simulink model "GuidanSim"  (R2024b)
settings: Solver=FixedStepAuto  StartTime=0.0  StopTime=inf  RelTol=1e-3
values from neighbouring files (symbols this model uses):
  gM = deg2rad(30)    [GuidanceSimParams.m]
  N = 2    [GuidanceSimParams.m]
  Rlethal = 1    [GuidanceSimParams.m]
  RM = [xM;zM]    [GuidanceSimParams.m]
  RT = [xT;zT]    [GuidanceSimParams.m]
  VM = [600*cos(gM),-600*sin(gM)]    [GuidanceSimParams.m]
  VT = [400*cos(gT),-400*sin(gT)]    [GuidanceSimParams.m]
libraries: simulink_extras x3, simulink x2, aerolibanim x1
settings Model: Creator=Ameya  LastModifiedBy=Ameya

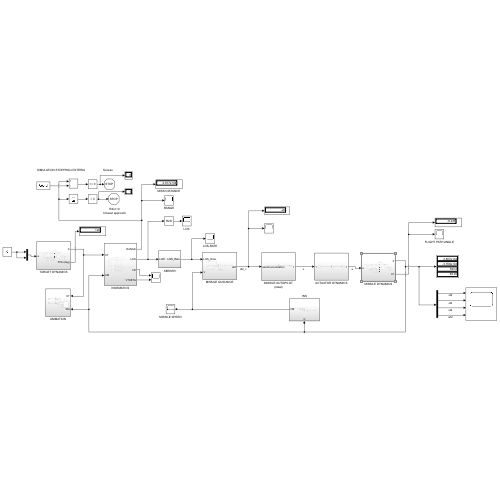
[thumbnail: Simulink's stored preview of the top-level diagram]
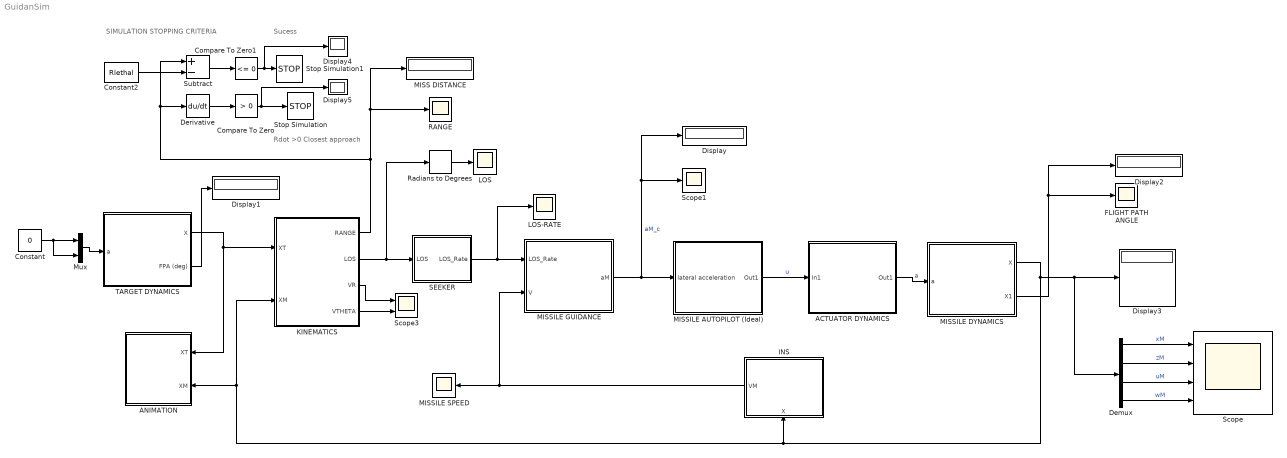
== system GuidanSim ==
  note: Rdot >0
      | Closest approach
  note: SIMULATION STOPPING CRITERIA
  note: Sucess
  ACTUATOR DYNAMICS : Subsystem
  ANIMATION : Subsystem
  Compare To Zero : simulink/Logic and Bit Operations/Compare To Zero  relop=>  OutDataTypeStr=boolean
  Compare To Zero1 : simulink/Logic and Bit Operations/Compare To Zero  relop=<=  OutDataTypeStr=boolean
  Constant : Constant  Value=0
  Constant2 : Constant  Value=Rlethal
  Demux : Demux
  Derivative : Derivative
  Display{,1..5} (6 alike) : Display
  FLIGHT PATH ANGLE : Scope
  INS : Subsystem
      settings: PortSchema="{\"entries\":[{\"content\":{\"sides\":[{\"content\":{},\"type\":\"ConnectorPlacement.EquallySpacedRectSide\",\"uuid\":\"3a75d8bd-203c-4ca4-9f28-a00dd574f861\"},{\"content\":{\"connectorIds\":[\"Out1\"],\"side\":\"RIGHT\"},\"type\":\"ConnectorPlacement.EquallySpacedRectSide\",\"uuid\":\"f6d8c757-0e96-437e-9198-94cbd887d432\"},{\"content\":{\"side\":\"TOP\"},\"type\":\"ConnectorPlacement.EquallySpacedRectSide\",\"uuid\":\"41075b2e-5d18-45ea-a6fc-7f66ef6598ab\"},{\"content\":{\"connectorIds\":[\"In1\"],\"side\":\"BOTTOM\"},\"type\":\"ConnectorPlacement.EquallySpacedRectSide\",\"uuid\":\"891ca2b5-b4ab-4086-9ff4-c4d2df822072\"}]},\"type\":\"ConnectorPlacement.EquallySpacedConnector\",\"uuid\":\"9a7247ef-0899-430c-baeb-b82ca1b0d294\"}],\"packageUris\":[\"http://schema.mathworks.com/mf0/Connector/R2020b\"],\"version\":\"1.0\"}"
  KINEMATICS : Subsystem
  LOS : Scope
  LOS-RATE : Scope
  MISS DISTANCE : Display
  MISSILE AUTOPILOT (Ideal) : Subsystem
  MISSILE DYNAMICS : Subsystem
  MISSILE GUIDANCE : Subsystem
  MISSILE SPEED : Scope
  Mux : Mux  Inputs=2
  RANGE : Scope
  Radians to Degrees : simulink_extras/Transformations/Radians to Degrees
  SEEKER : Subsystem
  Scope : Scope  NumInputPorts=4
  Scope1 : Scope
  Scope3 : Scope  NumInputPorts=2
  Stop Simulation : Stop
  Stop Simulation1 : Stop
  Subtract : Sum  Inputs=+-
  TARGET DYNAMICS : Subsystem
  wires:
  MISSILE AUTOPILOT (Ideal)/1(Out1) -> ACTUATOR DYNAMICS/1(In1)  "u"
  MISSILE GUIDANCE/1(aM) -> Scope1/1, Display/1, MISSILE AUTOPILOT (Ideal)/1(lateral acceleration)  "aM_c"
  ACTUATOR DYNAMICS/1(Out1) -> MISSILE DYNAMICS/1(a)  "a"
  MISSILE DYNAMICS/1(X) -> Demux/1, Display3/1, KINEMATICS/2(XM), ANIMATION/2(XM), INS/1(X)
  TARGET DYNAMICS/1(X) -> KINEMATICS/1(XT), ANIMATION/1(XT)
  SEEKER/1(LOS_Rate) -> LOS-RATE/1, MISSILE GUIDANCE/1(LOS_Rate)
  Constant/1 -> Mux/2, Mux/1
  Mux/1 -> TARGET DYNAMICS/1(a)
  KINEMATICS/2(LOS) -> Radians to Degrees/1, SEEKER/1(LOS)
  Radians to Degrees/1 -> LOS/1
  Compare To Zero/1 -> Display5/1, Stop Simulation/1
  Derivative/1 -> Compare To Zero/1
  KINEMATICS/1(RANGE) -> MISS DISTANCE/1, RANGE/1, Subtract/1, Derivative/1
  Constant2/1 -> Subtract/2
  Subtract/1 -> Compare To Zero1/1
  Compare To Zero1/1 -> Display4/1, Stop Simulation1/1
  INS/1(VM) -> MISSILE GUIDANCE/2(V), MISSILE SPEED/1
  Demux/1 -> Scope/1  "xM"
  Demux/2 -> Scope/2  "zM"
  Demux/3 -> Scope/3  "uM"
  Demux/4 -> Scope/4  "wM"
  KINEMATICS/3(VR) -> Scope3/1
  KINEMATICS/4(VTHETA) -> Scope3/2
  TARGET DYNAMICS/2(FPA (deg)) -> Display1/1
  MISSILE DYNAMICS/2(X1) -> Display2/1, FLIGHT PATH ANGLE/1

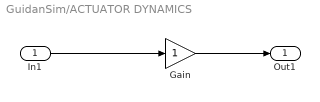
== system GuidanSim/ACTUATOR DYNAMICS ==
  In1 : Inport
  Gain : Gain
  Out1 : Outport
  wires:
  In1/1 -> Gain/1
  Gain/1 -> Out1/1

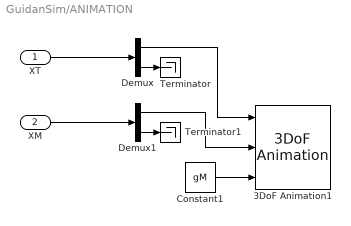
== system GuidanSim/ANIMATION ==
  XT : Inport
  XM : Inport  Port=2
  3DoF Animation1 : aerolibanim/3DoF Animation  u1=[0 5000 -2000 2000 -5050 -3]  u2=0.05  u3=5  u5=Fixed position  u6=[2000 500 -3150]  u7=10  u8=on
  Constant1 : Constant  Value=gM
  Demux : Demux  Outputs=2
  Demux1 : Demux  Outputs=2
  Terminator : Terminator
  Terminator1 : Terminator
  wires:
  Demux1/1 -> 3DoF Animation1/2
  XT/1 -> Demux/1
  Constant1/1 -> 3DoF Animation1/3
  Demux1/2 -> Terminator1/1
  Demux/1 -> 3DoF Animation1/1
  Demux/2 -> Terminator/1
  XM/1 -> Demux1/1

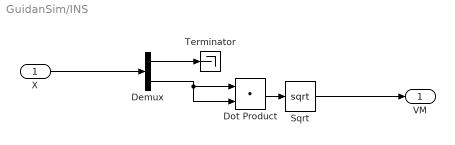
== system GuidanSim/INS ==
  X : Inport
  Demux : Demux  Outputs=2
  Dot Product : DotProduct  OutDataTypeStr=Inherit: Inherit via internal rule
  Sqrt : Sqrt
  Terminator : Terminator
  VM : Outport
  wires:
  X/1 -> Demux/1
  Demux/1 -> Terminator/1
  Dot Product/1 -> Sqrt/1
  Demux/2 -> Dot Product/1, Dot Product/2
  Sqrt/1 -> VM/1

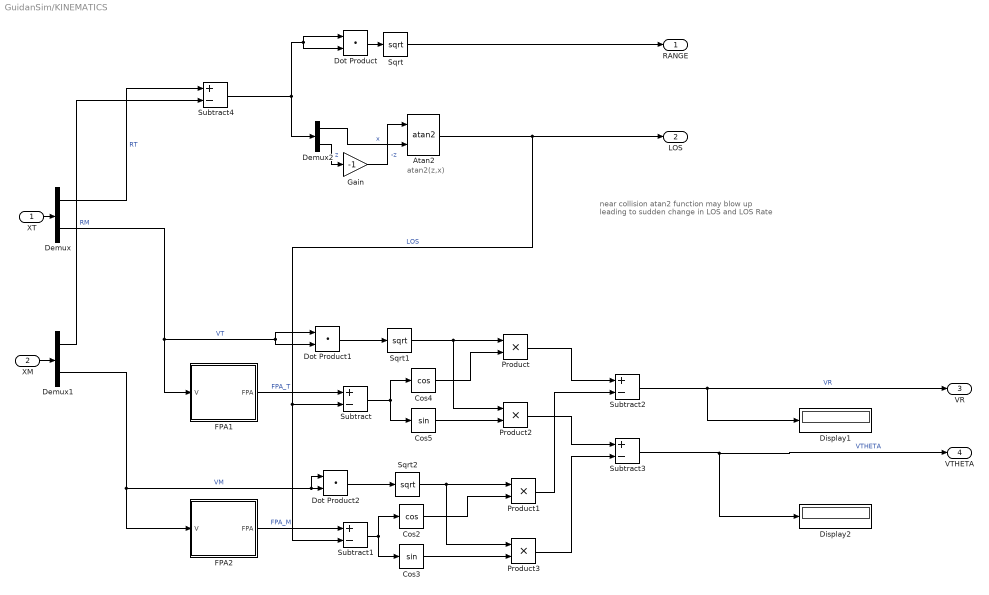
== system GuidanSim/KINEMATICS ==
  note: near collision atan2 function may blow up
      | leading to sudden change in LOS and LOS Rate
  note: atan2(z,x)
  XT : Inport
  XM : Inport  Port=2
  Atan2 : Trigonometry  Operator=atan2
  Cos2 : Trigonometry  Operator=cos
  Cos3 : Trigonometry
  Cos4 : Trigonometry  Operator=cos
  Cos5 : Trigonometry
  Demux : Demux  Outputs=2
  Demux1 : Demux  Outputs=2
  Demux2 : Demux  Outputs=2
  Display1 : Display
  Display2 : Display
  Dot Product : DotProduct  OutDataTypeStr=Inherit: Inherit via internal rule
  Dot Product1 : DotProduct  OutDataTypeStr=Inherit: Inherit via internal rule
  Dot Product2 : DotProduct  OutDataTypeStr=Inherit: Inherit via internal rule
  FPA1 : Subsystem
  FPA2 : Subsystem
  Gain : Gain  Gain=-1
  Product{,1..3} (4 alike) : Product
  Sqrt : Sqrt
  Sqrt1 : Sqrt
  Sqrt2 : Sqrt
  Subtract{,1..4} (5 alike) : Sum  Inputs=+-
  RANGE : Outport
  LOS : Outport  Port=2
  VR : Outport  Port=3
  VTHETA : Outport  Port=4
  wires:
  XT/1 -> Demux/1
  XM/1 -> Demux1/1
  Atan2/1 -> LOS/1, Subtract/2, Subtract1/2  "LOS"
  Demux/1 -> Subtract4/1  "RT"
  Demux1/1 -> Subtract4/2  "RM"
  Demux/2 -> Dot Product1/1, Dot Product1/2, FPA1/1(V)  "VT"
  FPA1/1(FPA) -> Subtract/1  "FPA_T"
  FPA2/1(FPA) -> Subtract1/1  "FPA_M"
  Subtract1/1 -> Cos3/1, Cos2/1
  Subtract/1 -> Cos5/1, Cos4/1
  Dot Product1/1 -> Sqrt1/1
  Sqrt1/1 -> Product2/1, Product/1
  Cos4/1 -> Product/2
  Sqrt2/1 -> Product3/1, Product1/1
  Demux1/2 -> Dot Product2/1, Dot Product2/2, FPA2/1(V)  "VM"
  Dot Product2/1 -> Sqrt2/1
  Cos2/1 -> Product1/2
  Product/1 -> Subtract2/1
  Product1/1 -> Subtract2/2
  Subtract2/1 -> VR/1, Display1/1  "VR"
  Subtract3/1 -> VTHETA/1, Display2/1  "VTHETA"
  Cos5/1 -> Product2/2
  Cos3/1 -> Product3/2
  Product3/1 -> Subtract3/2
  Product2/1 -> Subtract3/1
  Sqrt/1 -> RANGE/1
  Dot Product/1 -> Sqrt/1
  Gain/1 -> Atan2/1  "-z"
  Demux2/2 -> Gain/1  "z"
  Demux2/1 -> Atan2/2  "x"
  Subtract4/1 -> Dot Product/1, Dot Product/2, Demux2/1

== system GuidanSim/MISSILE AUTOPILOT (Ideal) ==
  lateral acceleration : Inport
  Gain : Gain
  Out1 : Outport
  wires:
  lateral acceleration/1 -> Gain/1
  Gain/1 -> Out1/1

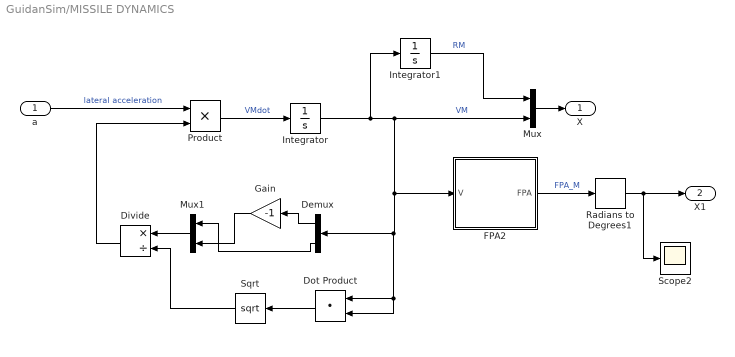
== system GuidanSim/MISSILE DYNAMICS ==
  a : Inport
  Demux : Demux  Outputs=2
  Divide : Product  Inputs=*/
  Dot Product : DotProduct  OutDataTypeStr=Inherit: Inherit via internal rule
  FPA2 : Subsystem
  Gain : Gain  Gain=-1
  Integrator : Integrator  InitialCondition=VM  UpperSaturationLimit=VM  LowerSaturationLimit=VM-0.000001
  Integrator1 : Integrator  InitialCondition=RM
  Mux : Mux  Inputs=2
  Mux1 : Mux  Inputs=2
  Product : Product
  Radians to Degrees1 : simulink_extras/Transformations/Radians to Degrees
  Scope2 : Scope
  Sqrt : Sqrt
  X : Outport
  X1 : Outport  Port=2
  wires:
  Integrator/1 -> Integrator1/1, FPA2/1(V), Dot Product/2, Dot Product/1, Demux/1, Mux/2  "VM"
  Integrator1/1 -> Mux/1  "RM"
  Mux/1 -> X/1
  Demux/1 -> Gain/1
  Gain/1 -> Mux1/2
  Demux/2 -> Mux1/1
  Dot Product/1 -> Sqrt/1
  a/1 -> Product/1  "lateral acceleration"
  Product/1 -> Integrator/1  "VMdot"
  Mux1/1 -> Divide/1
  Sqrt/1 -> Divide/2
  Divide/1 -> Product/2
  Radians to Degrees1/1 -> X1/1, Scope2/1
  FPA2/1(FPA) -> Radians to Degrees1/1  "FPA_M"

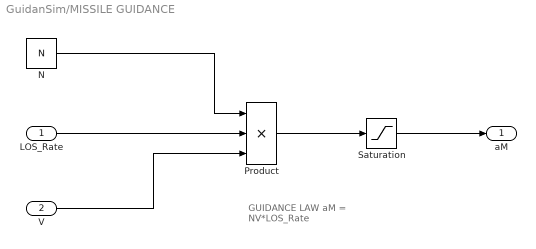
== system GuidanSim/MISSILE GUIDANCE ==
  note: GUIDANCE LAW
      | aM = NV*LOS_Rate
  LOS_Rate : Inport
  V : Inport  Port=2
  N : Constant  Value=N
  Product : Product  Inputs=3
  Saturation : Saturate  UpperLimit=+20  LowerLimit=-20
  aM : Outport
  wires:
  N/1 -> Product/1
  Product/1 -> Saturation/1
  LOS_Rate/1 -> Product/2
  V/1 -> Product/3
  Saturation/1 -> aM/1

== system GuidanSim/SEEKER ==
  LOS : Inport
  Derivative : Derivative
  LOS_Rate : Outport
  wires:
  LOS/1 -> Derivative/1
  Derivative/1 -> LOS_Rate/1

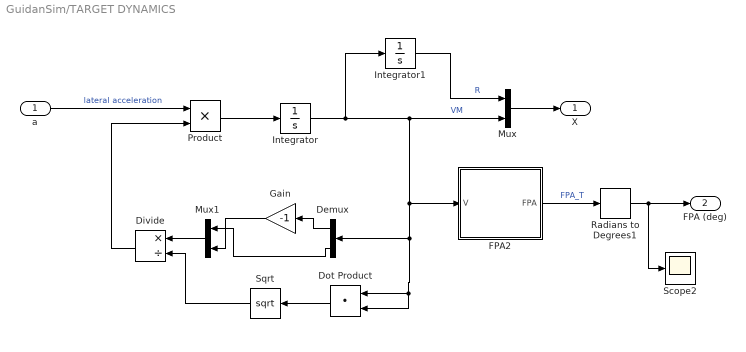
== system GuidanSim/TARGET DYNAMICS ==
  a : Inport
  Demux : Demux  Outputs=2
  Divide : Product  Inputs=*/
  Dot Product : DotProduct  OutDataTypeStr=Inherit: Inherit via internal rule
  FPA2 : Subsystem
  Gain : Gain  Gain=-1
  Integrator : Integrator  InitialCondition=VT
  Integrator1 : Integrator  InitialCondition=RT
  Mux : Mux  Inputs=2
  Mux1 : Mux  Inputs=2
  Product : Product
  Radians to Degrees1 : simulink_extras/Transformations/Radians to Degrees
  Scope2 : Scope
  Sqrt : Sqrt
  X : Outport
  FPA (deg) : Outport  Port=2
  wires:
  a/1 -> Product/1  "lateral acceleration"
  Integrator1/1 -> Mux/1  "R"
  Mux/1 -> X/1
  Demux/2 -> Mux1/1
  Dot Product/1 -> Sqrt/1
  Demux/1 -> Gain/1
  Sqrt/1 -> Divide/2
  Divide/1 -> Product/2
  Mux1/1 -> Divide/1
  Gain/1 -> Mux1/2
  Product/1 -> Integrator/1
  Integrator/1 -> Integrator1/1, FPA2/1(V), Dot Product/2, Dot Product/1, Demux/1, Mux/2  "VM"
  Radians to Degrees1/1 -> FPA (deg)/1, Scope2/1
  FPA2/1(FPA) -> Radians to Degrees1/1  "FPA_T"

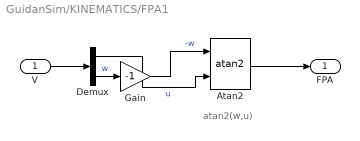
== system GuidanSim/KINEMATICS/FPA1 ==
  note: atan2(w,u)
  V : Inport
  Atan2 : Trigonometry  Operator=atan2
  Demux : Demux  Outputs=2
  Gain : Gain  Gain=-1
  FPA : Outport
  wires:
  V/1 -> Demux/1
  Demux/2 -> Gain/1  "w"
  Demux/1 -> Atan2/2  "u"
  Atan2/1 -> FPA/1
  Gain/1 -> Atan2/1  "-w"

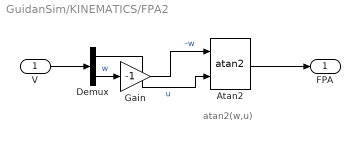
== system GuidanSim/KINEMATICS/FPA2 ==
  note: atan2(w,u)
  V : Inport
  Atan2 : Trigonometry  Operator=atan2
  Demux : Demux  Outputs=2
  Gain : Gain  Gain=-1
  FPA : Outport
  wires:
  V/1 -> Demux/1
  Demux/2 -> Gain/1  "w"
  Demux/1 -> Atan2/2  "u"
  Atan2/1 -> FPA/1
  Gain/1 -> Atan2/1  "-w"

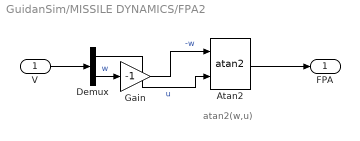
== system GuidanSim/MISSILE DYNAMICS/FPA2 ==
  note: atan2(w,u)
  V : Inport
  Atan2 : Trigonometry  Operator=atan2
  Demux : Demux  Outputs=2
  Gain : Gain  Gain=-1
  FPA : Outport
  wires:
  V/1 -> Demux/1
  Demux/2 -> Gain/1  "w"
  Demux/1 -> Atan2/2  "u"
  Atan2/1 -> FPA/1
  Gain/1 -> Atan2/1  "-w"

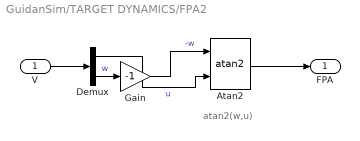
== system GuidanSim/TARGET DYNAMICS/FPA2 ==
  note: atan2(w,u)
  V : Inport
  Atan2 : Trigonometry  Operator=atan2
  Demux : Demux  Outputs=2
  Gain : Gain  Gain=-1
  FPA : Outport
  wires:
  V/1 -> Demux/1
  Demux/2 -> Gain/1  "w"
  Demux/1 -> Atan2/2  "u"
  Atan2/1 -> FPA/1
  Gain/1 -> Atan2/1  "-w"
